simulink model "model"  (R2024b)
settings: Solver=ode45  StartTime=0.0  StopTime=10  FixedStep=1e-6  MaxStep=1e-3  RelTol=1e-3  EnableMultiTasking=on
settings Model: Creator=rafac  LastModifiedBy=gmspe
settings SolverCC: AlgebraicLoopSolver=TrustRegion
settings DataIOCC: LimitDataPoints=on  SaveFormat=StructureWithTime  ReturnWorkspaceOutputs=off
settings OptimizationCC: LifeSpan=inf
settings DebuggingCC: FcnCallInpInsideContextMsg=warning  UnconnectedInputMsg=warning  UnconnectedOutputMsg=warning  UnconnectedLineMsg=warning  SFUnexpectedBacktrackingDiag=warning  SFNoUnconditionalDefaultTransitionDiag=warning  SFExecutionAtInitializationDiag=none  ArithmeticOperatorsInVariantConditions=warning
settings HardwareCC: ProdBitPerSizeT=32  ProdBitPerPtrDiffT=32  ProdWordSize=32  ProdHWDeviceType=Specified
settings ModelReferenceCC: PropagateSignalLabelsOutOfModel=off
settings SFSimCC: SimUseLocalCustomCode=off  CustomCodeUndefinedFunction=UseInterfaceOnly
settings RTWCC: RTWUseLocalCustomCode=off  GPUComputeCapability=3.5
settings CodeAppCC: StateflowObjectComments=on
settings GRTTargetCC: TargetLangStandard=C89/C90 (ANSI)
settings ConfigComp: CovMetricSettings=dw  CovSaveCumulativeToWorkspaceVar=on  CovSaveSingleToWorkspaceVar=on  CovExternalEMLEnable=off

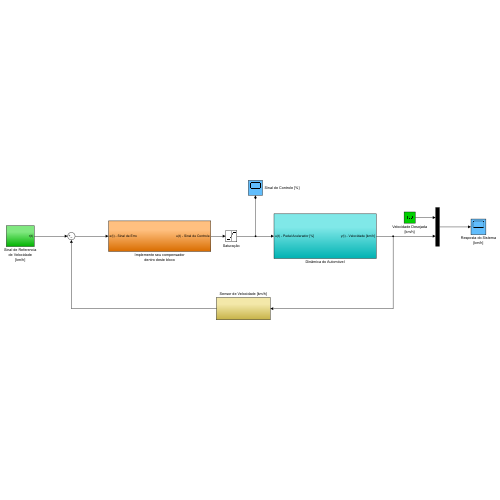
[thumbnail: Simulink's stored preview of the top-level diagram]
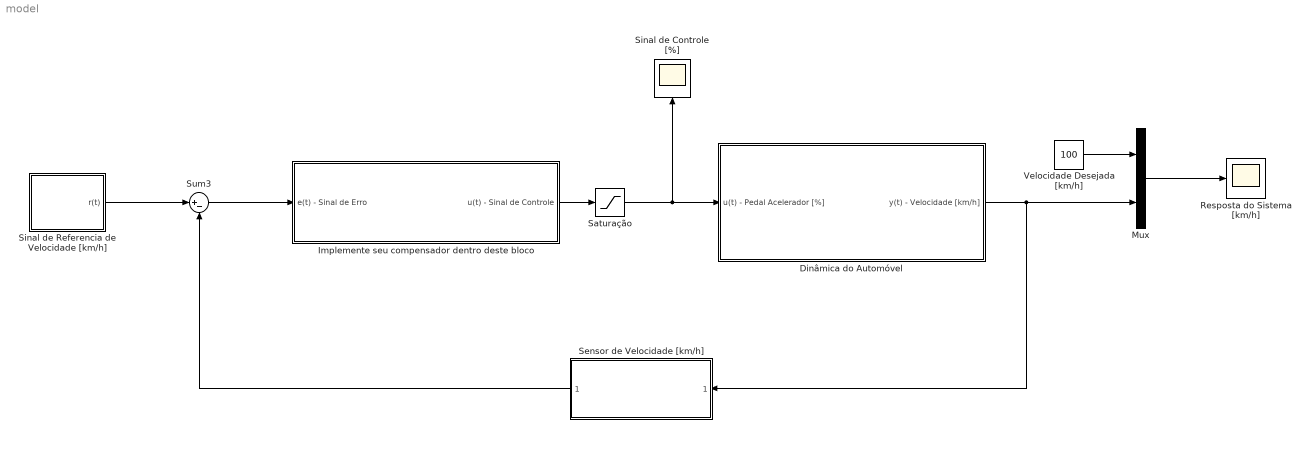
== system model ==
  Dinâmica do Automóvel : Subsystem
  Implemente seu compensador dentro deste bloco : Subsystem
  Mux : Mux  Inputs=2
  "Resposta do Sistema [km/h] " : Scope
  Saturação : Saturate  UpperLimit=100  LowerLimit=0
  Sensor de Velocidade [km/h] : Subsystem
  Sinal de Controle [%] : Scope
  Sinal de Referencia de Velocidade [km/h] : Subsystem
  Sum3 : Sum  Inputs=|+-
  Velocidade Desejada [km/h] : Constant  Value=100
  wires:
  Dinâmica do Automóvel/1(y(t) - Velocidade [km/h]) -> Mux/2, Sensor de Velocidade [km/h]/1("  ")
  Mux/1 -> "Resposta do Sistema [km/h] "/1
  Implemente seu compensador dentro deste bloco/1(u(t) - Sinal de Controle) -> Saturação/1
  Sum3/1 -> Implemente seu compensador dentro deste bloco/1(e(t) - Sinal de Erro)
  Saturação/1 -> Dinâmica do Automóvel/1(u(t) - Pedal Acelerador [%]), Sinal de Controle [%]/1
  Sensor de Velocidade [km/h]/1(" ") -> Sum3/2
  Sinal de Referencia de Velocidade [km/h]/1(r(t)) -> Sum3/1
  Velocidade Desejada [km/h]/1 -> Mux/1

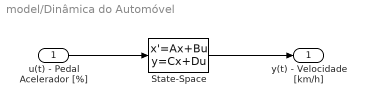
== system model/Dinâmica do Automóvel ==
  u(t) - Pedal Acelerador [%] : Inport
  State-Space : StateSpace  A=|  B=|  C="[1  0]"  D=0  InitialCondition=[80;0]
      A=|
      | [0 1
      | ; -c -b]
      B=|
      | [ 0
      |  ;  a ]
  y(t) - Velocidade [km/h] : Outport
  wires:
  State-Space/1 -> y(t) - Velocidade [km/h]/1
  u(t) - Pedal Acelerador [%]/1 -> State-Space/1

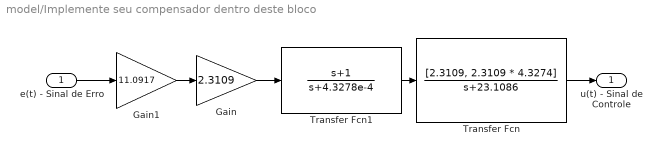
== system model/Implemente seu compensador dentro deste bloco ==
  e(t) - Sinal de Erro : Inport
  Gain : Gain  Gain=2.3109
  Gain1 : Gain  Gain=11.0917
  Transfer Fcn : TransferFcn  Numerator=[2.3109, 2.3109 * 4.3274]  Denominator=[1, 23.1086]
  Transfer Fcn1 : TransferFcn  Numerator=[1, 1]  Denominator=[1, 4.3278e-4]
  u(t) - Sinal de Controle : Outport
  wires:
  e(t) - Sinal de Erro/1 -> Gain1/1
  Gain1/1 -> Gain/1
  Gain/1 -> Transfer Fcn1/1
  Transfer Fcn1/1 -> Transfer Fcn/1
  Transfer Fcn/1 -> u(t) - Sinal de Controle/1

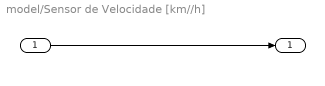
== system model/Sensor de Velocidade [km//h] ==
  "  " : Inport
  " " : Outport
  wires:
  "  "/1 -> " "/1

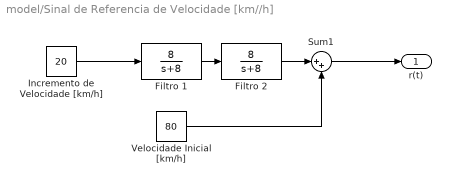
== system model/Sinal de Referencia de Velocidade [km//h] ==
  Filtro 1 : TransferFcn  Numerator=[8]  Denominator=[1 8]
  Filtro 2 : TransferFcn  Numerator=[8]  Denominator=[1 8]
  Incremento de Velocidade [km/h] : Constant  Value=20
  Sum1 : Sum  Inputs=|++
  Velocidade Inicial [km/h] : Constant  Value=80
  r(t) : Outport
  wires:
  Sum1/1 -> r(t)/1
  Filtro 1/1 -> Filtro 2/1
  Velocidade Inicial [km/h]/1 -> Sum1/2
  Incremento de Velocidade [km/h]/1 -> Filtro 1/1
  Filtro 2/1 -> Sum1/1
